simulink model "CM700A_HwTq3Meas"  (R2013b)
settings: Solver=FixedStepDiscrete  SolverMode=SingleTasking  StartTime=0.0  StopTime=1  FixedStep=0.002  RelTol=1e-3
values from neighbouring files (symbols this model uses):
  ELECGLBPRM_HWTQOFFS_HWNWTMTR_F32 = DataDict.Constant    [CM700A_HwTq3Meas_DataDict.m]
  ELECGLBPRM_HWTQSATNLOWRLIM_HWNWTMTR_F32 = DataDict.Constant    [CM700A_HwTq3Meas_DataDict.m]
  ELECGLBPRM_HWTQSATNUPPRLIM_HWNWTMTR_F32 = DataDict.Constant    [CM700A_HwTq3Meas_DataDict.m]
  ELECGLBPRM_HWTQSCA_ULS_F32 = DataDict.Constant    [CM700A_HwTq3Meas_DataDict.m]
  ELECGLBPRM_NOFLT_CNT_U08 = DataDict.Constant    [CM700A_HwTq3Meas_DataDict.m]
  ELECGLBPRM_OFFSTRIMNOTPRFM_CNT_U08 = DataDict.Constant    [CM700A_HwTq3Meas_DataDict.m]
  ELECGLBPRM_PRTCLFLT_CNT_U08 = DataDict.Constant    [CM700A_HwTq3Meas_DataDict.m]
  ELECGLBPRM_SNSRINTFLT_CNT_U08 = DataDict.Constant    [CM700A_HwTq3Meas_DataDict.m]
  GearIdn2 = DataDict.OpSignal    [CM700A_HwTq3Meas_DataDict.m]
  HwTq3MeasHwTq3PrtclFltFailStep = DataDict.Calibration    [CM700A_HwTq3Meas_DataDict.m]
  HwTq3MeasHwTq3PrtclFltPassStep = DataDict.Calibration    [CM700A_HwTq3Meas_DataDict.m]
undefined symbols (not defined in the file or in its folder): NtcNr1, NtcSts1, sigbuilder_block, SigQlfr1
libraries: simulink x22, NxtrNvM x3
(part 1 of 3)
settings Model: RequirementInfo={'doors' '00006115' '1' 'false' 'DOORS Surrogate Item' '' } %GIDa_184d7b6b_0c7e_41d3_b9a0_1a88eb3981d4  reqMgrSettings="100 S'doors','misc'{{S'surrogatepath','savemodel','savesurrogate','updateLinks','doorsLinks2sl','slLinks2Doors','purgeDoors','purgeSimulink','detaillevel','surrogateId','synctime'{{T\"/ESG Group/CM660A_HwTq1Meas\",M[1],M[1],M[0],M[0],M[1],M[0],M[0],M[1],T\"00006115\",T\"\"}},S'mode','pathStorage'{{T\"generic\",T\"modelRelative\"}}}}"  RecordCoverage=on  CovMetricSettings=dcmtrzoiw  CovFilter=CM700A_HwTq3Meas_covfilter  CovHTMLOptions=-sRT=1 -aTS=1 -bRG=1 -bTC=1 -hTR=0 -nFC=0 -scm=1 -bcm=1 -xEv=0  CovModelRefEnable=all  CovExternalEMLEnable=on  Creator=CZ68DS  LastModifiedBy=TZBSJD
settings SolverCC: AutoInsertRateTranBlk=on  InsertRTBMode=Always
settings DataIOCC: LimitDataPoints=off  SaveFormat=Structure  ReturnWorkspaceOutputs=on
settings OptimizationCC: BlockReduction=off  InlineParams=on  ZeroExternalMemoryAtStartup=off  ZeroInternalMemoryAtStartup=off  OptimizeModelRefInitCode=on  LifeSpan=1
settings DebuggingCC: SignalInfNanChecking=error  SignalRangeChecking=warning  UnderspecifiedInitializationDetection=Simplified  SolverPrmCheckMsg=error  InheritedTsInSrcMsg=error  DiscreteInheritContinuousMsg=error  SingleTaskRateTransMsg=error  TasksWithSamePriorityMsg=error  SigSpecEnsureSampleTimeMsg=error  CheckMatrixSingularityMsg=error  ParameterUnderflowMsg=error  ParameterPrecisionLossMsg=error  ParameterTunabilityLossMsg=error  FixptConstUnderflowMsg=warning  FixptConstOverflowMsg=warning  VectorMatrixConversionMsg=error  SignalLabelMismatchMsg=error  UnconnectedInputMsg=error  UnconnectedOutputMsg=error  UnconnectedLineMsg=error  SFcnCompatibilityMsg=error  UniqueDataStoreMsg=warning  BusObjectLabelMismatch=error  RootOutportRequireBusObject=error  AssertControl=DisableAll  ModelReferenceIOMsg=error  ModelReferenceVersionMismatchMessage=warning  ModelReferenceIOMismatchMessage=error  ModelReferenceCSMismatchMessage=warning  ModelReferenceDataLoggingMessage=error  StateNameClashWarn=warning  StrictBusMsg=ErrorOnBusTreatedAsVector  NonBusSignalsTreatedAsBus=error  SFUnexpectedBacktrackingDiag=error  SFInvalidInputDataAccessInChartInitDiag=error  SFNoUnconditionalDefaultTransitionDiag=error  SFTransitionOutsideNaturalParentDiag=error  SFUnconditionalTransitionShadowingDiag=error  SFUndirectedBroadcastEventsDiag=error
settings ModelReferenceCC: ModelReferenceNumInstancesAllowed=Single
settings RTWCC: SystemTargetFile=autosar.tlc  GenCodeOnly=on  TemplateMakefile=ert_default_tmf  Description=AUTOSAR  GenerateReport=on  ProcessScript=autosar_make_rtw_hook  LaunchReport=on
settings CodeAppCC: GenerateComments=off  IgnoreCustomStorageClasses=off  CustomSymbolStrType=$N$R$M  CustomSymbolStrBlkIO=$N$M  SimulinkBlockComments=off
settings STFCustomTargetCC: ParMdlRefBuildCompliant=on  CompOptLevelCompliant=on  IncludeMdlTerminateFcn=off  CombineOutputUpdateFcns=on  SuppressErrorStatus=on  ERTFirstTimeCompliant=on  ERTCustomFileBanners=on  SupportNonFinite=off  SupportComplex=off  SupportContinuousTime=off  SupportNonInlinedSFcns=off  MATLABClassNameForMDSCustomization=Simulink.SoftwareTarget.ERTCustomization  AutosarCompliant=on  GRTInterface=off  SystemTargetFile=autosar.tlc
settings ERTTargetCC: CodeReplacementLibrary=ANSI_C  ConcurrentExecutionCompliant=off  IncludeMdlTerminateFcn=off  SuppressErrorStatus=on  SupportNonFinite=off  SupportComplex=off  ModelStepFunctionPrototypeControlCompliant=off  CPPClassGenCompliant=off  AutosarCompliant=on  InlinedParameterPlacement=NonHierarchical  ERTCustomFileTemplate=example_file_process.tlc  EnableUserReplacementTypes=on

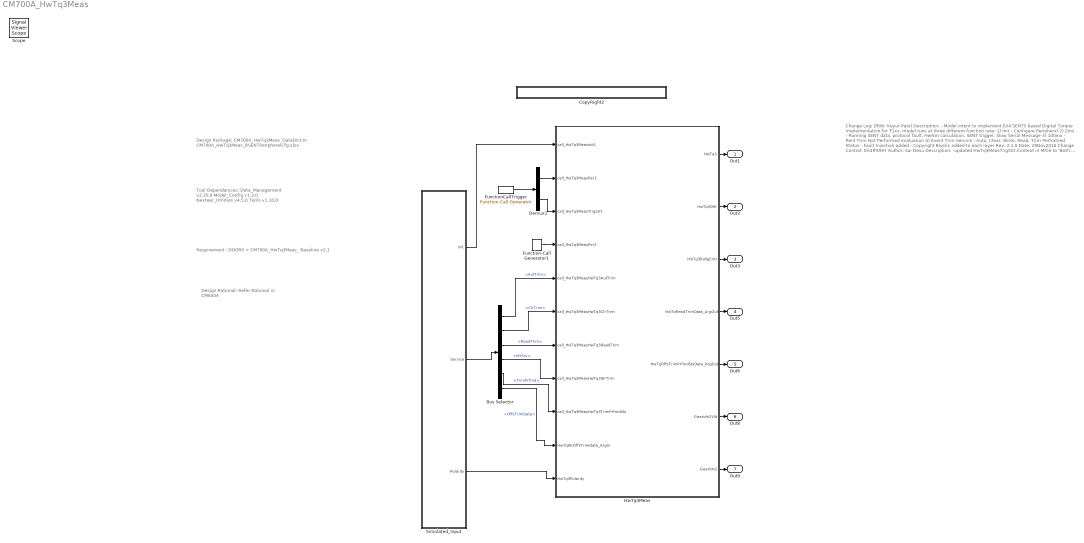
== system CM700A_HwTq3Meas ==
  note: Design Package:
      |
      | CM700A_HwTq3Meas_DataDict.m
      | CM700A_HwTq3Meas_RSENTPeripheralCfg.xlsx
  note: Change Log:
      |
      | DRW: Keyur Patel
      | Description:
      | - Model intent to implement EA4 SENT5 based Digital Torque implementation for T1xx.
      |    model runs at three different function rate:
      |       1) Init - Configure Peripheral
      |       2) 2ms - Running SENT data, protocol fault, HwNm calculation, SENT trigger, Slow Serial Message
      |       3) 100ms - Per3 Trim Not Performed evaluation
      |       4) Event Trim Service - Auto, Clear, Write, Read, Trim Performed Status
      | - Fault Injection added
      | - Copyright Blocks added to each layer
      |
      | Rev: 2.1.0
      | Date: 29Nov2016
      | Change Control: EA4#8597
      | Author: Sai Desu
      | Description:
      | -updated HwTq3MeasTrigStrt.Context in Mfile to 'Both'
      | -Removed Physical Inputs and Outputs from Mfile
      | -Grounded physical inputs and terminated Physical outputs in the model.
      |
      | Rev: 2.0.1
      | Date: 17MAY2016
      | Change Control: EA4#5776
      | Author: K. Patel
      | Description:
      | - GearIdn Uppler Limit and Lower Limit Added
      |
      |
      | Rev: 2.0.0
      | Date: 16MAR2016
      | Change Control: EA4#4736
      | Author: K. Patel
      | Description:
      | - Slow Serial Data Read Added for "C Factor & Bushing" signal read
      | - Timer 2us added before SPCT in NRS check added instead of SYNCM
      | - Refer Red Color High lighted Changes.
      |
      | Rev1.4.0
      | Date: 19JAN2016
      | Change Control #: 3378
      | DRW: K. Patel
      | Description:
      | - Refer Red Color High lighted Changes.
      | - "CM700A_HwTq3Meas_RSENTPeripheralCfg.xlsx" change
      |
      | Rev1.3.0
      | Date: 16DEC2015
      | Change Control #: 3161
      | DRW: K. Patel
      | Description:
      | - Refer Red Color High lighted Changes.
      |
      | Rev: 1.2.0
      | Date: 09OCT2015
      | Change Control #: EA4#1925
      | DRW: K. Patel
      | Description:
      | - Torque Trigger server function, Per3 change to Per2, Missing Message Counter add per1,
      | remove register from "CM700A_HwTq3Meas_RSENTPeripheralCfg.xlsx", change sync time to 16
      |
      | Rev: 1.1.0
      | Date: 31JUL2015
      | Change Control #: WCR-EA4#1232
      | DRW: K. Patel
      | Description:
      | - m file correction, Tick Time change from 1us to 1.2us
      | - Global Constant
      |
      | Rev: 1.0.0
      | Date: 06JUL2015
      | Change Control #: WCR-EA4#1033
      | DRW: K. Patel
      | Description:
      | - Initial Release
      | - Trim Services Added
  note: Tool Dependancies:
      |
      | Data_Management v2.35.0
      | Model_Config v1.3.0
      | Nexteer_Utilities v4.5.0
      | Tools v1.10.0
  note: Requirement :
      |
      | DOORS > CM700A_HwTq3Meas_ Baseline v2.1
  note: Design Rational:
      |
      | Refer Rational in CM650A
  Bus Selector : BusSelector  OutputSignals=AutTrim,ClrTrim,ReadTrim,WrSrv,TrimPrfmd,OffsTrimData
  CopyRight2 : Subsystem  Description=|  mask(Copyright Information){none=on}
      | Copyright info block.                                               
      |                                                                     
      | Place copyright information at the top of every subsystem in design.
      mask prompts: none "No parameters"
      mask help: Place copyright information at the top of every subsystem in design.
      mask Display:
      | NxtrConf = 'Nexteer Confidential';
      | 
      | sys = bdroot; %handle for the current model ("system")
      | first = get_param(sys,'Created');
      | first = first(end-3:end);  %year is last four digits
      | 
      | last = get_param(sys,'LastModifiedDate');
      | if isempty(last)
      |     last = datestr(now,'yyyy');
      | else
      |     last = last(end-3:end);
      | end
      | 
      | if strcmp(first,last)
      |     fprintf('%s -- Copyright %s Nexteer',NxtrConf,first)
      | else
      |     fprintf('%s -- %s%s- %s Nexteer',NxtrConf,char(169),first,last)
      | end
  Demux1 : Demux  Outputs=2
  Function-Call Generator1 : simulink/Ports & Subsystems/Function-Call Generator  sample_time=0.100  numberOfIterations=1
  FunctionCallTrigger : simulink/Ports & Subsystems/Function-Call Generator  RequirementInfo={} %GIDa_461051ca_e299_4da2_91c0_e73e41056377  sample_time=0.002  numberOfIterations=1
  HwTq3Meas : Subsystem  RequirementInfo={} %GIDa_76d712c1_5f1a_450e_83af_7c4f481758f4  Priority=1
      settings: AttributesFormatString=Priority = %<Priority>
  Simulated_Input : Subsystem  Description=Do not Code this block
      settings: AttributesFormatString=%<Description>
  Out1 : Outport
  Out2 : Outport  Port=2
  Out3 : Outport  Port=3
  Out5 : Outport  Port=4
  Out6 : Outport  Port=5
  Out8 : Outport  Port=6
  Out9 : Outport  Port=7
  Scope : SignalViewerScope  IOType=viewer  RefreshTime=0.035000
  wires:
  FunctionCallTrigger/1 -> Demux1/1
  Simulated_Input/3(Polarity) -> HwTq3Meas/11(HwTq3Polarity)
  HwTq3Meas/3(HwTq3RollgCntr) -> Out3/1
  HwTq3Meas/1(HwTq3) -> Out1/1
  HwTq3Meas/2(HwTq3Qlfr) -> Out2/1
  Function-Call Generator1/1 -> HwTq3Meas/4(call_HwTq3MeasPer2)
  Demux1/1 -> HwTq3Meas/2(call_HwTq3MeasPer1)
  Demux1/2 -> HwTq3Meas/3(call_HwTq3MeasTrigStrt)
  Bus Selector/1 -> HwTq3Meas/5(call_HwTq3MeasHwTq3AutTrim)  "<AutTrim>"
  Bus Selector/2 -> HwTq3Meas/6(call_HwTq3MeasHwTq3ClrTrim)  "<ClrTrim>"
  Bus Selector/3 -> HwTq3Meas/7(call_HwTq3MeasHwTq3ReadTrim)  "<ReadTrim>"
  Bus Selector/4 -> HwTq3Meas/8(call_HwTq3MeasHwTq3WrTrim)  "<WrSrv>"
  Bus Selector/5 -> HwTq3Meas/9(call_HwTq3MeasHwTq3TrimPrfmdSts)  "<TrimPrfmd>"
  Bus Selector/6 -> HwTq3Meas/10(HwTqWrOffsTrimData_ArgIn)  "<OffsTrimData>"
  Simulated_Input/1(Init) -> HwTq3Meas/1(call_HwTq3MeasInit1)
  Simulated_Input/2(Service) -> Bus Selector/1
  HwTq3Meas/4(HwTqReadTrimData_ArgOut) -> Out5/1
  HwTq3Meas/5(HwTqOffsTrimPrfmdStsData_ArgOut) -> Out6/1
  HwTq3Meas/6(GearIdn2Vld) -> Out8/1
  HwTq3Meas/7(GearIdn2) -> Out9/1

== system CM700A_HwTq3Meas/CopyRight2 ==

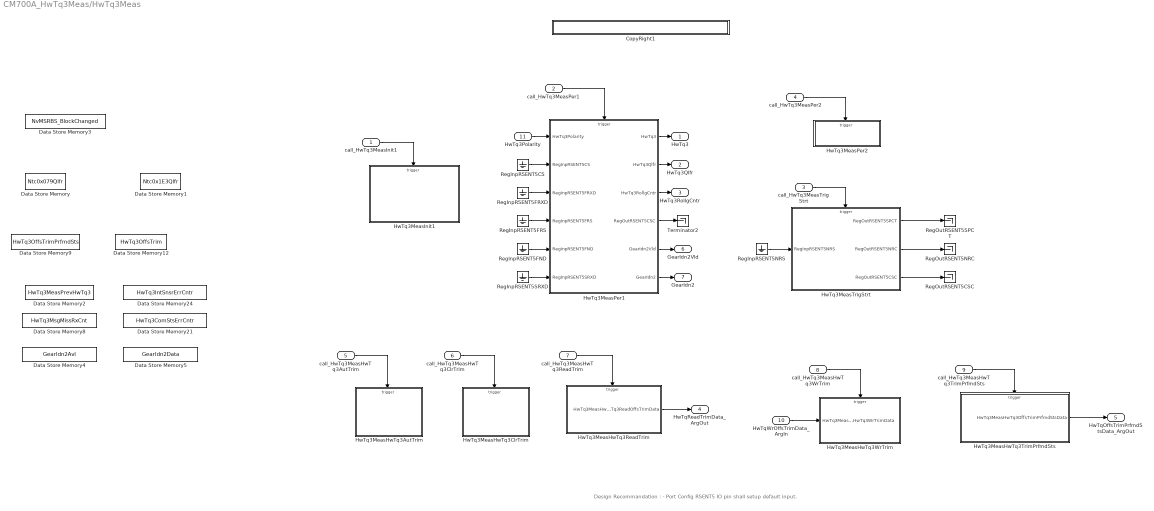
== system CM700A_HwTq3Meas/HwTq3Meas ==
  note: Design Recommandation :
      |
      | - Port Config RSENT5 IO pin shall setup default input.
  call_HwTq3MeasInit1 : Inport
  call_HwTq3MeasPer1 : Inport  Description=2ms  Port=2
      settings: AttributesFormatString=%<Description>
  call_HwTq3MeasTrigStrt : Inport  Description=Event  Port=3
      settings: AttributesFormatString=%<Description>
  call_HwTq3MeasPer2 : Inport  Description=100ms  Port=4
      settings: AttributesFormatString=%<Description>
  call_HwTq3MeasHwTq3AutTrim : Inport  Description=Event  Port=5
      settings: AttributesFormatString=%<Description>
  call_HwTq3MeasHwTq3ClrTrim : Inport  Description=Event  Port=6
      settings: AttributesFormatString=%<Description>
  call_HwTq3MeasHwTq3ReadTrim : Inport  Description=Event  Port=7
      settings: AttributesFormatString=%<Description>
  call_HwTq3MeasHwTq3WrTrim : Inport  Description=Event  Port=8
      settings: AttributesFormatString=%<Description>
  call_HwTq3MeasHwTq3TrimPrfmdSts : Inport  Description=Event  Port=9
      settings: AttributesFormatString=%<Description>
  HwTqWrOffsTrimData_ArgIn : Inport  Port=10
  HwTq3Polarity : Inport  Port=11  OutDataTypeStr=int8
  CopyRight1 : Subsystem  Description=|  mask(Copyright Information){none=on}
      | Copyright info block.                                               
      |                                                                     
      | Place copyright information at the top of every subsystem in design.
      mask prompts: none "No parameters"
      mask help: Place copyright information at the top of every subsystem in design.
      mask Display:
      | NxtrConf = 'Nexteer Confidential';
      | 
      | sys = bdroot; %handle for the current model ("system")
      | first = get_param(sys,'Created');
      | first = first(end-3:end);  %year is last four digits
      | 
      | last = get_param(sys,'LastModifiedDate');
      | if isempty(last)
      |     last = datestr(now,'yyyy');
      | else
      |     last = last(end-3:end);
      | end
      | 
      | if strcmp(first,last)
      |     fprintf('%s -- Copyright %s Nexteer',NxtrConf,first)
      | else
      |     fprintf('%s -- %s%s- %s Nexteer',NxtrConf,char(169),first,last)
      | end
  Data Store Memory12 : DataStoreMemory  DataStoreName=HwTq3OffsTrim  ReadBeforeWriteMsg=warning  WriteAfterWriteMsg=warning  WriteAfterReadMsg=warning
  Data Store Memory2 : DataStoreMemory  DataStoreName=HwTq3MeasPrevHwTq3  ReadBeforeWriteMsg=warning  WriteAfterWriteMsg=warning  WriteAfterReadMsg=warning  StateMustResolveToSignalObject=on
  Data Store Memory21 : DataStoreMemory  DataStoreName=HwTq3ComStsErrCntr  ReadBeforeWriteMsg=warning  WriteAfterWriteMsg=warning  WriteAfterReadMsg=warning  StateMustResolveToSignalObject=on
  Data Store Memory24 : DataStoreMemory  DataStoreName=HwTq3IntSnsrErrCntr  ReadBeforeWriteMsg=warning  WriteAfterWriteMsg=warning  WriteAfterReadMsg=warning  StateMustResolveToSignalObject=on
  Data Store Memory4 : DataStoreMemory  DataStoreName=GearIdn2Avl  ReadBeforeWriteMsg=warning  WriteAfterWriteMsg=warning  WriteAfterReadMsg=warning  StateMustResolveToSignalObject=on
  Data Store Memory5 : DataStoreMemory  DataStoreName=GearIdn2Data  ReadBeforeWriteMsg=warning  WriteAfterWriteMsg=warning  WriteAfterReadMsg=warning  StateMustResolveToSignalObject=on
  Data Store Memory8 : DataStoreMemory  DataStoreName=HwTq3MsgMissRxCnt  ReadBeforeWriteMsg=warning  WriteAfterWriteMsg=warning  WriteAfterReadMsg=warning  StateMustResolveToSignalObject=on
  Data Store Memory9 : DataStoreMemory  DataStoreName=HwTq3OffsTrimPrfmdSts  ReadBeforeWriteMsg=warning  WriteAfterWriteMsg=warning  WriteAfterReadMsg=warning
  Data Store Memory : DataStoreMemory  DataStoreName=Ntc0x079Qlfr  ReadBeforeWriteMsg=warning  WriteAfterWriteMsg=warning  WriteAfterReadMsg=warning  OutDataTypeStr=uint8
      settings: AttributesFormatString=|
      | Simulation Purpose Only.
      | Do Not Code this block
      | Diagnostic Manager Owns this requirement
  Data Store Memory1 : DataStoreMemory  DataStoreName=Ntc0x1E3Qlfr  ReadBeforeWriteMsg=warning  WriteAfterWriteMsg=warning  WriteAfterReadMsg=warning  OutDataTypeStr=uint8
      settings: AttributesFormatString=|
      | Simulation Purpose Only.
      | Do Not Code this block
      | Diagnostic Manager Owns this requirement
  Data Store Memory3 : DataStoreMemory  DataStoreName=NvMSRBS_BlockChanged  ReadBeforeWriteMsg=warning  WriteAfterWriteMsg=warning  WriteAfterReadMsg=warning  OutDataTypeStr=uint8
      settings: AttributesFormatString=|
      | Simulation Purpose Only.
      | Do Not Code this block
      | Diagnostic Manager Owns this requirement
  HwTq3MeasHwTq3AutTrim : Subsystem  RequirementInfo={'linktype_rmi_doors' '0000cf43 (/ESG Group/FDD Module Requirements/EA4 Specific/CM700A_HwTq3Meas)' '#CM700A_56' 'true' 'REQ: CM700A_56' '' } %GIDa_78a0150d_b2b2_4893_8cf0_7a267cd87682  Priority=10  TreatAsAtomicUnit=on
      settings: AttributesFormatString=Priority=%<Priority>
  HwTq3MeasHwTq3ClrTrim : Subsystem  RequirementInfo={'linktype_rmi_doors' '0000cf43 (/ESG Group/FDD Module Requirements/EA4 Specific/CM700A_HwTq3Meas)' '#CM700A_54' 'true' 'REQ: CM700A_54' '' } %GIDa_9d8bf3ad_e540_4a5e_ad4c_eb940ac157ad  Priority=10  TreatAsAtomicUnit=on
      settings: AttributesFormatString=Priority=%<Priority>
  HwTq3MeasHwTq3ReadTrim : Subsystem  RequirementInfo={'linktype_rmi_doors' '0000cf43 (/ESG Group/FDD Module Requirements/EA4 Specific/CM700A_HwTq3Meas)' '#CM700A_52' 'true' 'REQ: CM700A_52' '' } %GIDa_4c78535b_9e38_436f_a670_46438fd62cfe  Priority=10  TreatAsAtomicUnit=on
      settings: AttributesFormatString=Priority=%<Priority>
  HwTq3MeasHwTq3TrimPrfmdSts : Subsystem  RequirementInfo={'linktype_rmi_doors' '0000cf43 (/ESG Group/FDD Module Requirements/EA4 Specific/CM700A_HwTq3Meas)' '#CM700A_53' 'true' 'REQ: CM700A_53' '' } %GIDa_05e70ef2_f8d5_471c_a4a3_b95d94c92180  Priority=10  TreatAsAtomicUnit=on
      settings: AttributesFormatString=Priority=%<Priority>
  HwTq3MeasHwTq3WrTrim : Subsystem  RequirementInfo={'linktype_rmi_doors' '0000cf43 (/ESG Group/FDD Module Requirements/EA4 Specific/CM700A_HwTq3Meas)' '#CM700A_55' 'true' 'REQ: CM700A_55' '' } %GIDa_58f23a20_9e17_4252_b727_77362ca5c7be  Priority=10  TreatAsAtomicUnit=on
      settings: AttributesFormatString=Priority=%<Priority>
  HwTq3MeasInit1 : Subsystem  TreatAsAtomicUnit=on
  HwTq3MeasPer1 : Subsystem  RequirementInfo={'linktype_rmi_doors' '0000cf43 (/ESG Group/FDD Module Requirements/EA4 Specific/CM700A_HwTq3Meas)' '#CM700A_39' 'true' 'REQ: CM700A_39' '' } %GIDa_31b3da74_5937_4fb2_b915_5c5c5e5711e7  TreatAsAtomicUnit=on
  HwTq3MeasPer2 : Subsystem  RequirementInfo={'linktype_rmi_doors' '0000cf43 (/ESG Group/FDD Module Requirements/EA4 Specific/CM700A_HwTq3Meas)' '#CM700A_61' 'true' 'REQ: CM700A_61' '' } %GIDa_c89b04b6_b4c1_41bf_b3f8_efad30b9fb82  Priority=8  TreatAsAtomicUnit=on
      settings: AttributesFormatString=Priority=%<Priority>
  HwTq3MeasTrigStrt : Subsystem  RequirementInfo={'linktype_rmi_doors' '0000cf43 (/ESG Group/FDD Module Requirements/EA4 Specific/CM700A_HwTq3Meas)' '#CM700A_33' 'true' 'REQ: CM700A_33' '' } %GIDa_ac2e4248_233e_47e7_8dc6_e55969fb5c4e  TreatAsAtomicUnit=on
  RegInpRSENT5CS : Ground
  RegInpRSENT5FND : Ground
  RegInpRSENT5FRS : Ground
  RegInpRSENT5FRXD : Ground
  RegInpRSENT5NRS : Ground
  RegInpRSENT5SRXD : Ground
  RegOutRSENT5CSC : Terminator
  RegOutRSENT5NRC : Terminator
  RegOutRSENT5SPCT : Terminator
  Terminator2 : Terminator
  HwTq3 : Outport
  HwTq3Qlfr : Outport  Port=2
  HwTq3RollgCntr : Outport  Port=3
  HwTqReadTrimData_ArgOut : Outport  Port=4
  HwTqOffsTrimPrfmdStsData_ArgOut : Outport  Port=5
  GearIdn2Vld : Outport  Port=6
  GearIdn2 : Outport  Port=7
  wires:
  call_HwTq3MeasPer1/1 -> HwTq3MeasPer1/Trigger
  call_HwTq3MeasInit1/1 -> HwTq3MeasInit1/Trigger
  HwTq3MeasPer1/1(HwTq3) -> HwTq3/1
  HwTq3MeasPer1/2(HwTq3Qlfr) -> HwTq3Qlfr/1
  HwTq3MeasPer1/3(HwTq3RollgCntr) -> HwTq3RollgCntr/1
  call_HwTq3MeasTrigStrt/1 -> HwTq3MeasTrigStrt/Trigger
  HwTq3Polarity/1 -> HwTq3MeasPer1/1(HwTq3Polarity)
  HwTq3MeasTrigStrt/1(RegOutRSENT5SPCT) -> RegOutRSENT5SPCT/1
  call_HwTq3MeasHwTq3AutTrim/1 -> HwTq3MeasHwTq3AutTrim/Trigger
  call_HwTq3MeasHwTq3ClrTrim/1 -> HwTq3MeasHwTq3ClrTrim/Trigger
  call_HwTq3MeasHwTq3ReadTrim/1 -> HwTq3MeasHwTq3ReadTrim/Trigger
  call_HwTq3MeasHwTq3WrTrim/1 -> HwTq3MeasHwTq3WrTrim/Trigger
  call_HwTq3MeasHwTq3TrimPrfmdSts/1 -> HwTq3MeasHwTq3TrimPrfmdSts/Trigger
  HwTqWrOffsTrimData_ArgIn/1 -> HwTq3MeasHwTq3WrTrim/1(HwTq3MeasHwTq3WrTrimData)
  HwTq3MeasHwTq3ReadTrim/1(HwTq3MeasHwTq3ReadOffsTrimData) -> HwTqReadTrimData_ArgOut/1
  HwTq3MeasHwTq3TrimPrfmdSts/1(HwTq3MeasHwTq3OffsTrimPrfmdStsData) -> HwTqOffsTrimPrfmdStsData_ArgOut/1
  call_HwTq3MeasPer2/1 -> HwTq3MeasPer2/Trigger
  RegInpRSENT5CS/1 -> HwTq3MeasPer1/2(RegInpRSENT5CS)
  RegInpRSENT5FRXD/1 -> HwTq3MeasPer1/3(RegInpRSENT5FRXD)
  RegInpRSENT5FRS/1 -> HwTq3MeasPer1/4(RegInpRSENT5FRS)
  RegInpRSENT5FND/1 -> HwTq3MeasPer1/5(RegInpRSENT5FND)
  HwTq3MeasTrigStrt/2(RegOutRSENT5NRC) -> RegOutRSENT5NRC/1
  HwTq3MeasTrigStrt/3(RegOutRSENT5CSC) -> RegOutRSENT5CSC/1
  RegInpRSENT5NRS/1 -> HwTq3MeasTrigStrt/1(RegInpRSENT5NRS)
  HwTq3MeasPer1/4(RegOutRSENT5CSC) -> Terminator2/1
  RegInpRSENT5SRXD/1 -> HwTq3MeasPer1/6(RegInpRSENT5SRXD)
  HwTq3MeasPer1/5(GearIdn2Vld) -> GearIdn2Vld/1
  HwTq3MeasPer1/6(GearIdn2) -> GearIdn2/1

== system CM700A_HwTq3Meas/Simulated_Input ==
  Bus Creator : BusCreator  Inputs=6
  CopyRight2 : Subsystem  Description=|  mask(Copyright Information){none=on}
      | Copyright info block.                                               
      |                                                                     
      | Place copyright information at the top of every subsystem in design.
      mask prompts: none "No parameters"
      mask help: Place copyright information at the top of every subsystem in design.
      mask Display:
      | NxtrConf = 'Nexteer Confidential';
      | 
      | sys = bdroot; %handle for the current model ("system")
      | first = get_param(sys,'Created');
      | first = first(end-3:end);  %year is last four digits
      | 
      | last = get_param(sys,'LastModifiedDate');
      | if isempty(last)
      |     last = datestr(now,'yyyy');
      | else
      |     last = last(end-3:end);
      | end
      | 
      | if strcmp(first,last)
      |     fprintf('%s -- Copyright %s Nexteer',NxtrConf,first)
      | else
      |     fprintf('%s -- %s%s- %s Nexteer',NxtrConf,char(169),first,last)
      | end
  Data Type Conversion1 : DataTypeConversion  OutDataTypeStr=int8
  Data Type Conversion6 : DataTypeConversion  OutDataTypeStr=single
  Rate Transition : RateTransition
  Signal Builder : Subsystem  Tag=STV Subsys  LoadFcn=sigbuilder_block('load');  StartFcn=sigbuilder_block('start');  StopFcn=sigbuilder_block('stop');  ClipboardFcn=sigbuilder_block('clipboard');  mask(Sigbuilder block){}
      mask help: Simulink:masks:SigbuilderBlock_MD
      mask init:
      | if ~strcmp(get_param(bdroot(gcbh),'SimulationStatus'),'stopped') tuvar = sigbuilder_block('maskInit'); end
      settings: CopyFcn=sigbuilder_block('copy');  DeleteFcn=sigbuilder_block('delete');  ModelCloseFcn=sigbuilder_block('modelClose');  PreSaveFcn=sigbuilder_block('preSave');  PauseFcn=sigbuilder_block('pause');  ContinueFcn=sigbuilder_block('continue');  NameChangeFcn=sigbuilder_block('namechange');  OpenFcn=sigbuilder_block('open',[56.4828 0 967.655 519.517 ]);  CloseFcn=sigbuilder_block('close');
      mask Display: plot(0, 0, 100, 100,[2, 2, 32, 32, 2], [68, 8, 8, 68, 68],[32, 2], [38, 38], [32, 19, 2],[53, 60, 44], [32, 17, 17, 2],[16, 16, 31, 31]);txt = getActiveGroup(gcbh);text(2, 100, txt,'verticalAlignment', 'top');
  Init : Outport
  Service : Outport  Port=2
  Polarity : Outport  Port=3
  wires:
  Signal Builder/8(Polarity) -> Data Type Conversion1/1  "Polarity"
  Signal Builder/1(InitTrg) -> Init/1
  Signal Builder/7(HwTqOffsTrimData) -> Data Type Conversion6/1
  Signal Builder/6(TrimPrfmdStsSrv) -> Bus Creator/5  "TrimPrfmd"
  Signal Builder/5(WrSrv) -> Bus Creator/4  "WrSrv"
  Signal Builder/4(ReadTrimSrv) -> Bus Creator/3  "ReadTrim"
  Signal Builder/3(ClearTrimSrv) -> Bus Creator/2  "ClrTrim"
  Signal Builder/2(AutTrimSrv) -> Bus Creator/1  "AutTrim"
  Bus Creator/1 -> Service/1
  Data Type Conversion1/1 -> Rate Transition/1
  Rate Transition/1 -> Polarity/1
  Data Type Conversion6/1 -> Bus Creator/6  "OffsTrimData"

== system CM700A_HwTq3Meas/HwTq3Meas/CopyRight1 ==

== system CM700A_HwTq3Meas/HwTq3Meas/HwTq3MeasHwTq3AutTrim ==
  function : TriggerPort
  CopyRight2 : Subsystem  Description=|  mask(Copyright Information){none=on}
      | Copyright info block.                                               
      |                                                                     
      | Place copyright information at the top of every subsystem in design.
      mask prompts: none "No parameters"
      mask help: Place copyright information at the top of every subsystem in design.
      mask Display:
      | NxtrConf = 'Nexteer Confidential';
      | 
      | sys = bdroot; %handle for the current model ("system")
      | first = get_param(sys,'Created');
      | first = first(end-3:end);  %year is last four digits
      | 
      | last = get_param(sys,'LastModifiedDate');
      | if isempty(last)
      |     last = datestr(now,'yyyy');
      | else
      |     last = last(end-3:end);
      | end
      | 
      | if strcmp(first,last)
      |     fprintf('%s -- Copyright %s Nexteer',NxtrConf,first)
      | else
      |     fprintf('%s -- %s%s- %s Nexteer',NxtrConf,char(169),first,last)
      | end
  NVM Shadow RAM : DataStoreWrite  RequirementInfo={} %GIDa_691c2588_2b45_48b9_9733_fd18f25444bb  DataStoreName=HwTq3OffsTrim
  NVM1 Shadow RAM : DataStoreWrite  RequirementInfo={'linktype_rmi_doors' '0000cf43 (/ESG Group/FDD Module Requirements/EA4 Specific/CM700A_HwTq3Meas)' '#CM700A_50' 'true' 'REQ: CM700A_50' '' } %GIDa_8dfe2b68_c9bd_4b5f_9a85_4945a725dea6  DataStoreName=HwTq3OffsTrimPrfmdSts
  PIM : DataStoreRead  RequirementInfo={} %GIDa_7720d852_cab6_4ee8_822b_ee5ddb596286  Priority=10  DataStoreName=HwTq3MeasPrevHwTq3
      settings: AttributesFormatString=Priority=%<Priority>
  Set : Constant
  Set Ram Block Status : NxtrNvM/Set Ram Block Status  FuncName=Set Ram Block Status  NvMBlockName=HwTq3Offs  VoidFuncRtn=on  BlockChanged_DSN=NvMSRBS_BlockChanged  Return_DSN=NvMSRBS_Return
      settings: AttributesFormatString=%<FuncName>
  Set3 : Constant  OutDataTypeStr=uint8
  wires:
  PIM/1 -> NVM Shadow RAM/1
  Set/1 -> NVM1 Shadow RAM/1
  Set3/1 -> Set Ram Block Status/1

== system CM700A_HwTq3Meas/HwTq3Meas/HwTq3MeasHwTq3ClrTrim ==
  function : TriggerPort
  Clear1 : Constant  Value=0  OutDataTypeStr=single
  Clear2 : Constant  Value=0
  CopyRight2 : Subsystem  Description=|  mask(Copyright Information){none=on}
      | Copyright info block.                                               
      |                                                                     
      | Place copyright information at the top of every subsystem in design.
      mask prompts: none "No parameters"
      mask help: Place copyright information at the top of every subsystem in design.
      mask Display:
      | NxtrConf = 'Nexteer Confidential';
      | 
      | sys = bdroot; %handle for the current model ("system")
      | first = get_param(sys,'Created');
      | first = first(end-3:end);  %year is last four digits
      | 
      | last = get_param(sys,'LastModifiedDate');
      | if isempty(last)
      |     last = datestr(now,'yyyy');
      | else
      |     last = last(end-3:end);
      | end
      | 
      | if strcmp(first,last)
      |     fprintf('%s -- Copyright %s Nexteer',NxtrConf,first)
      | else
      |     fprintf('%s -- %s%s- %s Nexteer',NxtrConf,char(169),first,last)
      | end
  NVM Shadow RAM : DataStoreWrite  RequirementInfo={} %GIDa_c01938bd_873a_4f20_8aad_b7368db2e426  DataStoreName=HwTq3OffsTrim
  NVM1 Shadow RAM : DataStoreWrite  RequirementInfo={'linktype_rmi_doors' '0000cf43 (/ESG Group/FDD Module Requirements/EA4 Specific/CM700A_HwTq3Meas)' '#CM700A_50' 'true' 'REQ: CM700A_50' '' } %GIDa_7e661117_be14_43c5_b4c7_51bd14c3b186  DataStoreName=HwTq3OffsTrimPrfmdSts
  Set Ram Block Status : NxtrNvM/Set Ram Block Status  FuncName=Set Ram Block Status  NvMBlockName=HwTq3Offs  VoidFuncRtn=on  BlockChanged_DSN=NvMSRBS_BlockChanged  Return_DSN=NvMSRBS_Return
      settings: AttributesFormatString=%<FuncName>
  Set3 : Constant  OutDataTypeStr=uint8
  wires:
  Clear1/1 -> NVM Shadow RAM/1
  Clear2/1 -> NVM1 Shadow RAM/1
  Set3/1 -> Set Ram Block Status/1

== system CM700A_HwTq3Meas/HwTq3Meas/HwTq3MeasHwTq3ReadTrim ==
  function : TriggerPort
  CopyRight2 : Subsystem  Description=|  mask(Copyright Information){none=on}
      | Copyright info block.                                               
      |                                                                     
      | Place copyright information at the top of every subsystem in design.
      mask prompts: none "No parameters"
      mask help: Place copyright information at the top of every subsystem in design.
      mask Display:
      | NxtrConf = 'Nexteer Confidential';
      | 
      | sys = bdroot; %handle for the current model ("system")
      | first = get_param(sys,'Created');
      | first = first(end-3:end);  %year is last four digits
      | 
      | last = get_param(sys,'LastModifiedDate');
      | if isempty(last)
      |     last = datestr(now,'yyyy');
      | else
      |     last = last(end-3:end);
      | end
      | 
      | if strcmp(first,last)
      |     fprintf('%s -- Copyright %s Nexteer',NxtrConf,first)
      | else
      |     fprintf('%s -- %s%s- %s Nexteer',NxtrConf,char(169),first,last)
      | end
  NVM Shadow RAM : DataStoreRead  DataStoreName=HwTq3OffsTrim
  HwTq3MeasHwTq3ReadOffsTrimData : Outport
  wires:
  NVM Shadow RAM/1 -> HwTq3MeasHwTq3ReadOffsTrimData/1

== system CM700A_HwTq3Meas/HwTq3Meas/HwTq3MeasHwTq3TrimPrfmdSts ==
  function : TriggerPort
  CopyRight2 : Subsystem  Description=|  mask(Copyright Information){none=on}
      | Copyright info block.                                               
      |                                                                     
      | Place copyright information at the top of every subsystem in design.
      mask prompts: none "No parameters"
      mask help: Place copyright information at the top of every subsystem in design.
      mask Display:
      | NxtrConf = 'Nexteer Confidential';
      | 
      | sys = bdroot; %handle for the current model ("system")
      | first = get_param(sys,'Created');
      | first = first(end-3:end);  %year is last four digits
      | 
      | last = get_param(sys,'LastModifiedDate');
      | if isempty(last)
      |     last = datestr(now,'yyyy');
      | else
      |     last = last(end-3:end);
      | end
      | 
      | if strcmp(first,last)
      |     fprintf('%s -- Copyright %s Nexteer',NxtrConf,first)
      | else
      |     fprintf('%s -- %s%s- %s Nexteer',NxtrConf,char(169),first,last)
      | end
  Data Store Read1 : DataStoreRead  DataStoreName=HwTq3OffsTrimPrfmdSts
  HwTq3MeasHwTq3OffsTrimPrfmdStsData : Outport
  wires:
  Data Store Read1/1 -> HwTq3MeasHwTq3OffsTrimPrfmdStsData/1

== system CM700A_HwTq3Meas/HwTq3Meas/HwTq3MeasHwTq3WrTrim ==
  HwTq3MeasHwTq3WrTrimData : Inport
  function : TriggerPort
  CopyRight2 : Subsystem  Description=|  mask(Copyright Information){none=on}
      | Copyright info block.                                               
      |                                                                     
      | Place copyright information at the top of every subsystem in design.
      mask prompts: none "No parameters"
      mask help: Place copyright information at the top of every subsystem in design.
      mask Display:
      | NxtrConf = 'Nexteer Confidential';
      | 
      | sys = bdroot; %handle for the current model ("system")
      | first = get_param(sys,'Created');
      | first = first(end-3:end);  %year is last four digits
      | 
      | last = get_param(sys,'LastModifiedDate');
      | if isempty(last)
      |     last = datestr(now,'yyyy');
      | else
      |     last = last(end-3:end);
      | end
      | 
      | if strcmp(first,last)
      |     fprintf('%s -- Copyright %s Nexteer',NxtrConf,first)
      | else
      |     fprintf('%s -- %s%s- %s Nexteer',NxtrConf,char(169),first,last)
      | end
  NVM Shadow RAM : DataStoreWrite  RequirementInfo={} %GIDa_1659f01a_6b97_4ff1_afb0_e4ba99927e44  DataStoreName=HwTq3OffsTrim
  NVM1 Shadow RAM : DataStoreWrite  RequirementInfo={'linktype_rmi_doors' '0000cf43 (/ESG Group/FDD Module Requirements/EA4 Specific/CM700A_HwTq3Meas)' '#CM700A_50' 'true' 'REQ: CM700A_50' '' } %GIDa_340e34c7_c59a_43cb_a8d9_5aafb58ec96b  DataStoreName=HwTq3OffsTrimPrfmdSts
  Set : Constant
  Set Ram Block Status : NxtrNvM/Set Ram Block Status  FuncName=Set Ram Block Status  NvMBlockName=HwTq3Offs  VoidFuncRtn=on  BlockChanged_DSN=NvMSRBS_BlockChanged  Return_DSN=NvMSRBS_Return
      settings: AttributesFormatString=%<FuncName>
  Set3 : Constant  OutDataTypeStr=uint8
  wires:
  Set/1 -> NVM1 Shadow RAM/1
  HwTq3MeasHwTq3WrTrimData/1 -> NVM Shadow RAM/1
  Set3/1 -> Set Ram Block Status/1

== system CM700A_HwTq3Meas/HwTq3Meas/HwTq3MeasInit1 ==
  note: Follow below steps in same order:
      |
      | 1. Enable Configuration mode, RSENT5MDC.OMC = 1U
      | 2. Verify whether peripheral is in Configuration mode RSENT5MST.OMS ==1U and wait till 2us* ,it is in configuration mode
      | 3. Configure the SENT Register as per  "CM700A_HwTq3Meas_RSENTPeripheralCfg.xlsx"
      | 4. Enable Operation active mode, RSENT5MDC.OMC = 5U
      | 5. Verify whether peripheral is in Opertation active mode RSENT5MST.OMS ==5U and wait till 2us* ,it is in Opertation active mode
      | 6. Client Call "IoHwAb_SetFctPrphlHwTq3"- Port Configuration shall change to output in alternate mode from default input for RSENT5 SPCO IO pin.
      |
      | Note: * - actual minimum is 150ns as per Scott Winder email from Renesas
  function : TriggerPort  TriggerType=falling
  CopyRight2 : Subsystem  Description=|  mask(Copyright Information){none=on}
      | Copyright info block.                                               
      |                                                                     
      | Place copyright information at the top of every subsystem in design.
      mask prompts: none "No parameters"
      mask help: Place copyright information at the top of every subsystem in design.
      mask Display:
      | NxtrConf = 'Nexteer Confidential';
      | 
      | sys = bdroot; %handle for the current model ("system")
      | first = get_param(sys,'Created');
      | first = first(end-3:end);  %year is last four digits
      | 
      | last = get_param(sys,'LastModifiedDate');
      | if isempty(last)
      |     last = datestr(now,'yyyy');
      | else
      |     last = last(end-3:end);
      | end
      | 
      | if strcmp(first,last)
      |     fprintf('%s -- Copyright %s Nexteer',NxtrConf,first)
      | else
      |     fprintf('%s -- %s%s- %s Nexteer',NxtrConf,char(169),first,last)
      | end
  GetRefTmr1MicroSec32bit : Subsystem
      settings: AttributesFormatString=Client Call : Start Time
  GetTiSpan1MicroSec32bit : Subsystem
  IoHwAb_SetFctPrphlHwTq3 : Subsystem
  Terminator1 : Terminator
  wires:
  GetRefTmr1MicroSec32bit/1(RefTmr) -> GetTiSpan1MicroSec32bit/1(RefTmr)
  GetTiSpan1MicroSec32bit/1(TiSpan) -> Terminator1/1

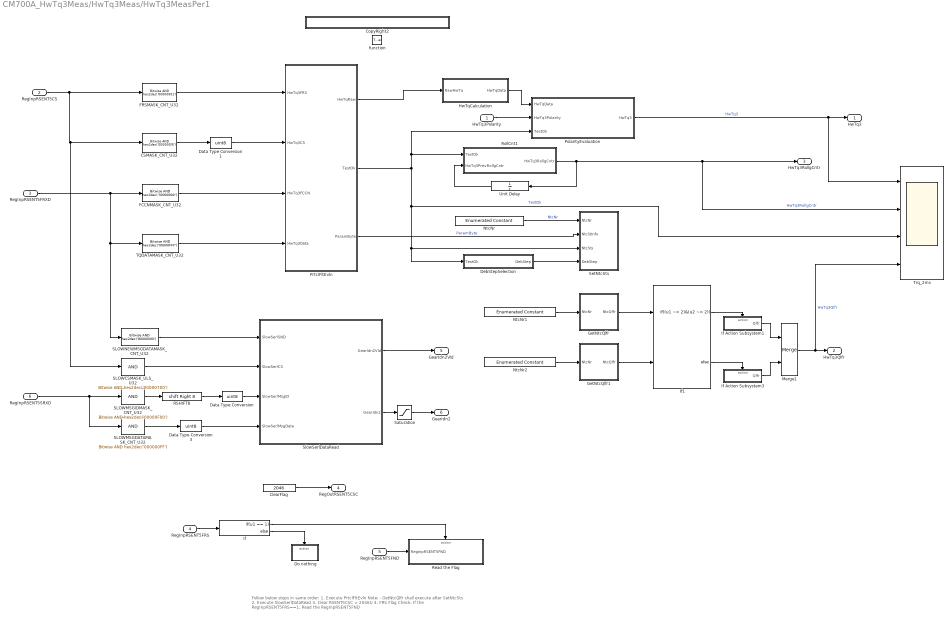
== system CM700A_HwTq3Meas/HwTq3Meas/HwTq3MeasPer1 ==
  note: Follow below steps in same order:
      |
      | 1. Execute PrtclFltEvln
      | Note: - GetNtcQlfr shall execute after SetNtcSts
      | 2. Execute SlowSerlDataRead
      | 3. Clear RSENT5CSC = 2046U
      | 4. FRS Flag Check: If the RegInpRSENT5FRS==1,  Read the RegInpRSENT5FND
  HwTq3Polarity : Inport
  RegInpRSENT5CS : Inport  Port=2
  RegInpRSENT5FRXD : Inport  Port=3
  RegInpRSENT5FRS : Inport  Port=4
  RegInpRSENT5FND : Inport  Port=5
  RegInpRSENT5SRXD : Inport  Port=6
  function : TriggerPort  TriggerType=function-call
  CSMASK_CNT_U32 : simulink/Logic and Bit Operations/Bitwise Operator  logicop=AND  UseBitMask=on  BitMask=hex2dec('000000FE')  BitMaskRealWorld=Stored Integer
  ClearFlag : Constant  RequirementInfo={} %GIDa_f85a4098_a822_4f75_a0b4_b2fef5bc9e6f  Value=2046  OutDataTypeStr=uint16
  CopyRight2 : Subsystem  Description=|  mask(Copyright Information){none=on}
      | Copyright info block.                                               
      |                                                                     
      | Place copyright information at the top of every subsystem in design.
      mask prompts: none "No parameters"
      mask help: Place copyright information at the top of every subsystem in design.
      mask Display:
      | NxtrConf = 'Nexteer Confidential';
      | 
      | sys = bdroot; %handle for the current model ("system")
      | first = get_param(sys,'Created');
      | first = first(end-3:end);  %year is last four digits
      | 
      | last = get_param(sys,'LastModifiedDate');
      | if isempty(last)
      |     last = datestr(now,'yyyy');
      | else
      |     last = last(end-3:end);
      | end
      | 
      | if strcmp(first,last)
      |     fprintf('%s -- Copyright %s Nexteer',NxtrConf,first)
      | else
      |     fprintf('%s -- %s%s- %s Nexteer',NxtrConf,char(169),first,last)
      | end
  Data Type Conversion : DataTypeConversion  OutDataTypeStr=uint8
  Data Type Conversion1 : DataTypeConversion  OutDataTypeStr=uint8
  Data Type Conversion3 : DataTypeConversion  OutDataTypeStr=uint8
  DebStepSelection : Subsystem
  Do nothing : Subsystem  RequirementInfo={} %GIDa_36aa72da_c0b3_4756_827c_f0dd9940ca90  TreatAsAtomicUnit=on
  FCCNMASK_CNT_U32 : simulink/Logic and Bit Operations/Bitwise Operator  logicop=AND  UseBitMask=on  BitMask=hex2dec('30000000')  BitMaskRealWorld=Stored Integer
  FRSMASK_CNT_U32 : simulink/Logic and Bit Operations/Bitwise Operator  logicop=AND  UseBitMask=on  BitMask=hex2dec('00000001')  BitMaskRealWorld=Stored Integer
  GetNtcQlfr : Subsystem
  GetNtcQlfr1 : Subsystem
  HwTqCalculation : Subsystem
  If : If  RequirementInfo={} %GIDa_9a3999db_ec42_4cbc_a179_526d044a0c5a  IfExpression=u1 == 1
  If Action Subsystem1 : Subsystem  TreatAsAtomicUnit=on
  If Action Subsystem3 : Subsystem  TreatAsAtomicUnit=on
  If1 : If  NumInputs=2  IfExpression=(u1 ~= 2)&(u2 ~= 2)
  Merge1 : Merge
  NtcNr : simulink/Sources/Enumerated Constant  OutDataTypeStr=Enum: NtcNr1  Value=NtcNr1.NTCNR_0X079  SampleTime=inf
  NtcNr1 : simulink/Sources/Enumerated Constant  OutDataTypeStr=Enum: NtcNr1  Value=NtcNr1.NTCNR_0X079  SampleTime=inf
  NtcNr2 : simulink/Sources/Enumerated Constant  OutDataTypeStr=Enum: NtcNr1  Value=NtcNr1.NTCNR_0X1E3  SampleTime=inf
  PolarityEvaluation : Subsystem  RequirementInfo={'linktype_rmi_doors' '0000cf43 (/ESG Group/FDD Module Requirements/EA4 Specific/CM700A_HwTq3Meas)' '#CM700A_29' 'true' 'REQ: CM700A_29' '' ; 'linktype_rmi_doors' '0000cf43 (/ESG Group/FDD Module Requirements/EA4 Specific/CM700A_HwTq3Meas)' '#CM700A_32' 'true' 'REQ: CM700A_32' '' } %GIDa_7dd0f124_da9d_41af_bfd5_c8f0b8205e28
  PrtclFltEvln : Subsystem  RequirementInfo={'doors' '00006115' '16' 'false' 'DOORS Surrogate Item' '' ; 'linktype_rmi_doors' '0000cf43 (/ESG Group/FDD Module Requirements/EA4 Specific/CM700A_HwTq3Meas)' '#CM700A_27' 'true' 'REQ: CM700A_27' '' } %GIDa_9ddede9b_2ee1_447b_ab8b_835557d5d4fb
  RSHIFT8 : ArithShift  BitShiftNumber=8  BitShiftDirection=Right
  Read the Flag : Subsystem  RequirementInfo={} %GIDa_8292da39_c813_49b3_bba8_7ea1e085c113  TreatAsAtomicUnit=on
  RollCnt1 : Stateflow chart  RequirementInfo={} %GIDa_be1c412e_1791_4e7e_9b3e_cc09ba9a6629  TreatAsAtomicUnit=on
  SLOWCSMASK_ULS_U32 : simulink/Logic and Bit Operations/Bitwise Operator  logicop=AND  UseBitMask=on  BitMask=hex2dec('00000700')  BitMaskRealWorld=Stored Integer
  SLOWMSGDATAMASK_CNT_U32 : simulink/Logic and Bit Operations/Bitwise Operator  logicop=AND  UseBitMask=on  BitMask=hex2dec('000000FF')  BitMaskRealWorld=Stored Integer
  SLOWMSGIDMASK_CNT_U32 : simulink/Logic and Bit Operations/Bitwise Operator  logicop=AND  UseBitMask=on  BitMask=hex2dec('00000F00')  BitMaskRealWorld=Stored Integer
  SLOWNEWMSGDATAMASK_CNT_U32 : simulink/Logic and Bit Operations/Bitwise Operator  logicop=AND  UseBitMask=on  BitMask=hex2dec('80000000')  BitMaskRealWorld=Stored Integer
  Saturation : Saturate  UpperLimit=GearIdn2.EngMax  LowerLimit=GearIdn2.EngMin
      settings: AttributesFormatString=|
      | %<LowerLimit>
      | %<UpperLimit>
  SetNtcSts : Subsystem  RequirementInfo={'linktype_rmi_doors' '0000cf43 (/ESG Group/FDD Module Requirements/EA4 Specific/CM700A_HwTq3Meas)' '#CM700A_38' 'true' 'REQ: CM700A_38' '' } %GIDa_7c28da3a_b49c_4a2c_9776_430afb4b2413
  SlowSerlDataRead : Subsystem  RequirementInfo={'linktype_rmi_doors' '0000cf43 (/ESG Group/FDD Module Requirements/EA4 Specific/CM700A_HwTq3Meas)' '#CM700A_66' 'true' 'REQ: CM700A_66' '' } %GIDa_a534ff24_7731_4575_902d_df9a309aff98
  TQDATAMASK_CNT_U32 : simulink/Logic and Bit Operations/Bitwise Operator  logicop=AND  UseBitMask=on  BitMask=hex2dec('00000FFF')  BitMaskRealWorld=Stored Integer
  Trq_2ms : Scope  NumInputPorts=4
      settings: TimeRange=20  YMin=-10~0~1.9~0.95  YMax=10~275~2.1~1.05  SaveName=ScopeData3
  Unit Delay : UnitDelay  SampleTime=-1  StateName=HwTq3MeasPrevRollgCntr  StateMustResolveToSignalObject=on
      settings: AttributesFormatString=%<StateName>
  HwTq3 : Outport  RequirementInfo={} %GIDa_3b2abd0f_dff5_44f3_b788_adb2172836f5
  HwTq3Qlfr : Outport  RequirementInfo={'linktype_rmi_doors' '0000cf43 (/ESG Group/FDD Module Requirements/EA4 Specific/CM700A_HwTq3Meas)' '#CM700A_30' 'true' 'REQ: CM700A_30' '' } %GIDa_5eff5979_1038_44df_a727_ac7fcfb158b0  Port=2
  HwTq3RollgCntr : Outport  RequirementInfo={'linktype_rmi_doors' '0000cf43 (/ESG Group/FDD Module Requirements/EA4 Specific/CM700A_HwTq3Meas)' '#CM700A_31' 'true' 'REQ: CM700A_31' '' } %GIDa_de83414f_64c7_40b0_8047_6b8baba686d2  Port=3
  RegOutRSENT5CSC : Outport  Port=4
  GearIdn2Vld : Outport  RequirementInfo={} %GIDa_d279c553_77c2_4307_9c21_10957e80324d  Port=5
  GearIdn2 : Outport  RequirementInfo={} %GIDa_0355680d_a243_40f6_8530_f1f9bdf0d0ac  Port=6
  wires:
  PrtclFltEvln/1(HwTqRaw) -> HwTqCalculation/1(RawHwTq)
  HwTqCalculation/1(HwTqData) -> PolarityEvaluation/1(HwTqData)
  PrtclFltEvln/2(TestOk) -> PolarityEvaluation/3(TestOk), RollCnt1/1(TestOk), Trq_2ms/3, SetNtcSts/3(NtcSts), DebStepSelection/1(TestOk)  "TestOk"
  HwTq3Polarity/1 -> PolarityEvaluation/2(HwTq3Polarity)
  NtcNr/1 -> SetNtcSts/1(NtcNr)  "NtcNr"
  PrtclFltEvln/3(ParamByte) -> SetNtcSts/2(NtcStInfo)  "ParamByte"
  NtcNr1/1 -> GetNtcQlfr/1(NtcNr)
  DebStepSelection/1(DebStep) -> SetNtcSts/4(DebStep)
  PolarityEvaluation/1(HwTq3) -> Trq_2ms/1, HwTq3/1  "HwTq3"
  RollCnt1/1(HwTq3RollgCntr) -> Unit Delay/1, Trq_2ms/2, HwTq3RollgCntr/1  "HwTq3RollgCntr"
  Unit Delay/1 -> RollCnt1/2(HwTq3PrevRollgCntr)
  NtcNr2/1 -> GetNtcQlfr1/1(NtcNr)
  GetNtcQlfr/1(NtcQlfr) -> If1/1
  GetNtcQlfr1/1(NtcQlfr) -> If1/2
  If Action Subsystem1/1(Qlfr) -> Merge1/1
  If Action Subsystem3/1(Qlfr) -> Merge1/2
  Merge1/1 -> Trq_2ms/4, HwTq3Qlfr/1  "HwTq3Qlfr"
  If1/2 -> If Action Subsystem3/Action
  If1/1 -> If Action Subsystem1/Action
  FCCNMASK_CNT_U32/1 -> PrtclFltEvln/3(HwTq3FCCN)
  TQDATAMASK_CNT_U32/1 -> PrtclFltEvln/4(HwTq3Data)
  RegInpRSENT5FRS/1 -> If/1
  If/1 -> Read the Flag/Action
  If/2 -> Do nothing/Action
  RegInpRSENT5FND/1 -> Read the Flag/1(RegInpRSENT5FND)
  ClearFlag/1 -> RegOutRSENT5CSC/1
  CSMASK_CNT_U32/1 -> Data Type Conversion1/1
  FRSMASK_CNT_U32/1 -> PrtclFltEvln/1(HwTq3FRS)
  Data Type Conversion1/1 -> PrtclFltEvln/2(HwTq3CS)
  RegInpRSENT5FRXD/1 -> SLOWNEWMSGDATAMASK_CNT_U32/1, TQDATAMASK_CNT_U32/1, FCCNMASK_CNT_U32/1
  RegInpRSENT5CS/1 -> SLOWCSMASK_ULS_U32/1, CSMASK_CNT_U32/1, FRSMASK_CNT_U32/1
  SlowSerlDataRead/1(GearIdn2Vld) -> GearIdn2Vld/1
  SlowSerlDataRead/2(GearIdn2) -> Saturation/1
  SLOWCSMASK_ULS_U32/1 -> SlowSerlDataRead/2(SlowSerlCS)
  SLOWNEWMSGDATAMASK_CNT_U32/1 -> SlowSerlDataRead/1(SlowSerlSND)
  RegInpRSENT5SRXD/1 -> SLOWMSGDATAMASK_CNT_U32/1, SLOWMSGIDMASK_CNT_U32/1
  SLOWMSGIDMASK_CNT_U32/1 -> RSHIFT8/1
  SLOWMSGDATAMASK_CNT_U32/1 -> Data Type Conversion3/1
  RSHIFT8/1 -> Data Type Conversion/1
  Data Type Conversion3/1 -> SlowSerlDataRead/4(SlowSerlMsgData)
  Data Type Conversion/1 -> SlowSerlDataRead/3(SlowSerlMsgID)
  Saturation/1 -> GearIdn2/1

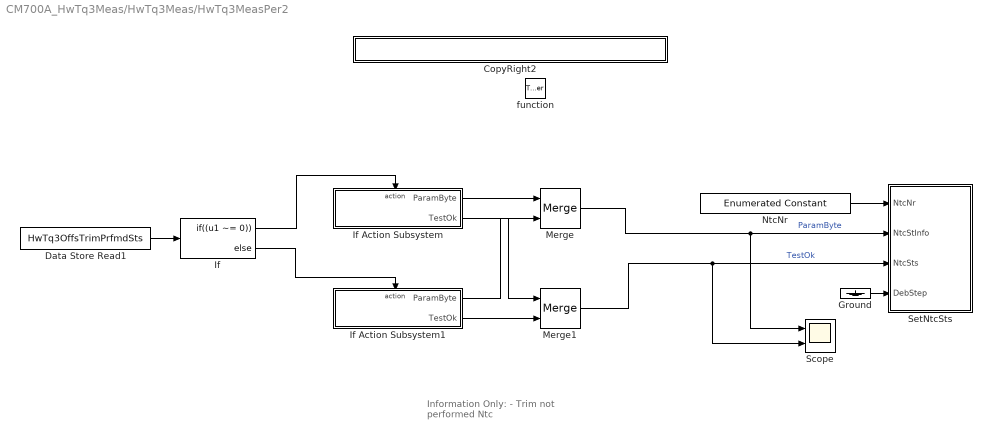
== system CM700A_HwTq3Meas/HwTq3Meas/HwTq3MeasPer2 ==
  note: Information Only:
      | - Trim not performed Ntc
  function : TriggerPort  TriggerType=function-call
  CopyRight2 : Subsystem  Description=|  mask(Copyright Information){none=on}
      | Copyright info block.                                               
      |                                                                     
      | Place copyright information at the top of every subsystem in design.
      mask prompts: none "No parameters"
      mask help: Place copyright information at the top of every subsystem in design.
      mask Display:
      | NxtrConf = 'Nexteer Confidential';
      | 
      | sys = bdroot; %handle for the current model ("system")
      | first = get_param(sys,'Created');
      | first = first(end-3:end);  %year is last four digits
      | 
      | last = get_param(sys,'LastModifiedDate');
      | if isempty(last)
      |     last = datestr(now,'yyyy');
      | else
      |     last = last(end-3:end);
      | end
      | 
      | if strcmp(first,last)
      |     fprintf('%s -- Copyright %s Nexteer',NxtrConf,first)
      | else
      |     fprintf('%s -- %s%s- %s Nexteer',NxtrConf,char(169),first,last)
      | end
  Data Store Read1 : DataStoreRead  DataStoreName=HwTq3OffsTrimPrfmdSts
  Ground : Ground
  If : If  IfExpression=(u1 ~= 0)
  If Action Subsystem : Subsystem  RequirementInfo={'linktype_rmi_doors' '0000cf43 (/ESG Group/FDD Module Requirements/EA4 Specific/CM700A_HwTq3Meas)' '#CM700A_65' 'true' 'REQ: CM700A_65' '' } %GIDa_eda0e9fe_0ef4_4d37_918c_815346a1604f  TreatAsAtomicUnit=on
  If Action Subsystem1 : Subsystem  RequirementInfo={'linktype_rmi_doors' '0000cf43 (/ESG Group/FDD Module Requirements/EA4 Specific/CM700A_HwTq3Meas)' '#CM700A_63' 'true' 'REQ: CM700A_63' '' } %GIDa_f1a05e9a_fff8_4eab_8b85_2e72f495a740  TreatAsAtomicUnit=on
  Merge : Merge
  Merge1 : Merge
  NtcNr : simulink/Sources/Enumerated Constant  OutDataTypeStr=Enum: NtcNr1  Value=NtcNr1.NTCNR_0X1E3  SampleTime=inf
  Scope : Scope  NumInputPorts=2
      settings: YMin=-5~-5  YMax=5~5  SaveName=ScopeData3
  SetNtcSts : Subsystem  RequirementInfo={'linktype_rmi_doors' '0000cf43 (/ESG Group/FDD Module Requirements/EA4 Specific/CM700A_HwTq3Meas)' '#CM700A_59' 'true' 'REQ: CM700A_59' '' } %GIDa_03dde2fd_062f_4b23_859a_fc5579118954
  wires:
  Ground/1 -> SetNtcSts/4(DebStep)
  NtcNr/1 -> SetNtcSts/1(NtcNr)
  Data Store Read1/1 -> If/1
  If/1 -> If Action Subsystem/Action
  If/2 -> If Action Subsystem1/Action
  If Action Subsystem/1(ParamByte) -> Merge/1
  If Action Subsystem1/1(ParamByte) -> Merge/2
  If Action Subsystem/2(TestOk) -> Merge1/1
  If Action Subsystem1/2(TestOk) -> Merge1/2
  Merge/1 -> Scope/1, SetNtcSts/2(NtcStInfo)  "ParamByte"
  Merge1/1 -> Scope/2, SetNtcSts/3(NtcSts)  "TestOk"

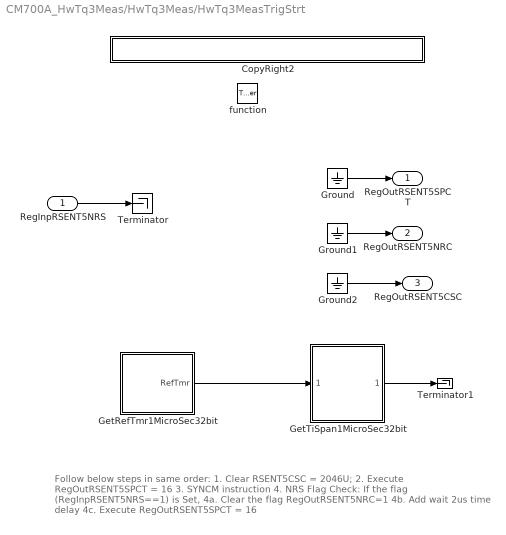
== system CM700A_HwTq3Meas/HwTq3Meas/HwTq3MeasTrigStrt ==
  note: Follow below steps in same order:
      |
      | 1. Clear RSENT5CSC = 2046U;
      | 2. Execute RegOutRSENT5SPCT = 16
      | 3. SYNCM instruction
      |
      | 4. NRS Flag Check: If the flag (RegInpRSENT5NRS==1) is Set,
      | 	4a. Clear the flag RegOutRSENT5NRC=1
      | 	4b. Add wait 2us time delay
      | 	4c. Execute RegOutRSENT5SPCT = 16
  RegInpRSENT5NRS : Inport
  function : TriggerPort  TriggerType=function-call
  CopyRight2 : Subsystem  Description=|  mask(Copyright Information){none=on}
      | Copyright info block.                                               
      |                                                                     
      | Place copyright information at the top of every subsystem in design.
      mask prompts: none "No parameters"
      mask help: Place copyright information at the top of every subsystem in design.
      mask Display:
      | NxtrConf = 'Nexteer Confidential';
      | 
      | sys = bdroot; %handle for the current model ("system")
      | first = get_param(sys,'Created');
      | first = first(end-3:end);  %year is last four digits
      | 
      | last = get_param(sys,'LastModifiedDate');
      | if isempty(last)
      |     last = datestr(now,'yyyy');
      | else
      |     last = last(end-3:end);
      | end
      | 
      | if strcmp(first,last)
      |     fprintf('%s -- Copyright %s Nexteer',NxtrConf,first)
      | else
      |     fprintf('%s -- %s%s- %s Nexteer',NxtrConf,char(169),first,last)
      | end
  GetRefTmr1MicroSec32bit : Subsystem
      settings: AttributesFormatString=Client Call : Start Time
  GetTiSpan1MicroSec32bit : Subsystem
  Ground : Ground
  Ground1 : Ground
  Ground2 : Ground
  Terminator : Terminator
  Terminator1 : Terminator
  RegOutRSENT5SPCT : Outport
  RegOutRSENT5NRC : Outport  Port=2
  RegOutRSENT5CSC : Outport  Port=3
  wires:
  Ground1/1 -> RegOutRSENT5NRC/1
  Ground/1 -> RegOutRSENT5SPCT/1
  Ground2/1 -> RegOutRSENT5CSC/1
  RegInpRSENT5NRS/1 -> Terminator/1
  GetTiSpan1MicroSec32bit/1(TiSpan) -> Terminator1/1
  GetRefTmr1MicroSec32bit/1(RefTmr) -> GetTiSpan1MicroSec32bit/1(RefTmr)

== system CM700A_HwTq3Meas/Simulated_Input/CopyRight2 ==

== system CM700A_HwTq3Meas/Simulated_Input/Signal Builder ==
  Demux : Demux  Tag=STV Demux  Outputs=8
  FromWs : FromWorkspace  Tag=STV FromWs  VariableName=tuvar  SampleTime=0  OutputAfterFinalValue=Holding final value
      SigBuilderData=|
      | common.afterFinalStr = 'Hold final value'
      | common.sampleTime = '0'
      | dataSet(1).timeRange = [0 20]
      | dataSet(1).name = 'IdealSignal'
      | dataSet(2).timeRange = [0 20]
      | dataSet(2).name = 'Faults'
      | dataSet(3).timeRange = [0 20]
      | dataSet(3).name = 'Service'
      | sbobj.Groups(1).Name = 'IdealSignal'
      | sbobj.Groups(1).Signals(1).Name = 'InitTrg'
      | sbobj.Groups(1).Signals(1).XData = [0 0.02 0.02 0.06 0.06 20]
      | sbobj.Groups(1).Signals(1).YData = [0 0 1 1 0 0]
      | sbobj.Groups(1).Signals(2).Name = 'AutTrimSrv'
      | sbobj.Groups(1).Signals(2).XData = [0 20]
      | sbobj.Groups(1).Signals(2).YData = [0 0]
      | sbobj.Groups(1).Signals(3).Name = 'ClearTrimSrv'
      | sbobj.Groups(1).Signals(3).XData = [0 20]
      | sbobj.Groups(1).Signals(3).YData = [0 0]
      | sbobj.Groups(1).Signals(4).Name = 'ReadTrimSrv'
      | sbobj.Groups(1).Signals(4).XData = [0 20]
      | sbobj.Groups(1).Signals(4).YData = [0 0]
      | sbobj.Groups(1).Signals(5).Name = 'WrSrv'
      | sbobj.Groups(1).Signals(5).XData = [0 0.04 0.04 0.08 0.08 20]
      | sbobj.Groups(1).Signals(5).YData = [0 0 1 1 0 0]
      | sbobj.Groups(1).Signals(6).Name = 'TrimPrfmdStsSrv'
      | sbobj.Groups(1).Signals(6).XData = [0 20]
      | sbobj.Groups(1).Signals(6).YData = [0 0]
      | sbobj.Groups(1).Signals(7).Name = 'HwTqOffsTrimData'
      | sbobj.Groups(1).Signals(7).XData = [0 20]
      | sbobj.Groups(1).Signals(7).YData = [0 0]
      | sbobj.Groups(1).Signals(8).Name = 'Polarity'
      | sbobj.Groups(1).Signals(8).XData = [0 20]
      | sbobj.Groups(1).Signals(8).YData = [1 1]
      | sbobj.Groups(1).TimeRange = [0 20]
      | sbobj.Groups(2).Name = 'Faults'
      | sbobj.Groups(2).Signals(1).Name = 'InitTrg'
      | sbobj.Groups(2).Signals(1).XData = [0 0.02 0.02 0.06 0.06 20]
      | sbobj.Groups(2).Signals(1).YData = [0 0 1 1 0 0]
      | sbobj.Groups(2).Signals(2).Name = 'AutTrimSrv'
      | sbobj.Groups(2).Signals(2).XData = [0 20]
      | sbobj.Groups(2).Signals(2).YData = [0 0]
      | sbobj.Groups(2).Signals(3).Name = 'ClearTrimSrv'
      | sbobj.Groups(2).Signals(3).XData = [0 20]
      | sbobj.Groups(2).Signals(3).YData = [0 0]
      | sbobj.Groups(2).Signals(4).Name = 'ReadTrimSrv'
      | sbobj.Groups(2).Signals(4).XData = [0 20]
      | sbobj.Groups(2).Signals(4).YData = [0 0]
      | sbobj.Groups(2).Signals(5).Name = 'WrSrv'
      | sbobj.Groups(2).Signals(5).XData = [0 0.06 0.06 0.12 0.12 20]
      | sbobj.Groups(2).Signals(5).YData = [0 0 1 1 0 0]
      | sbobj.Groups(2).Signals(6).Name = 'TrimPrfmdStsSrv'
      | sbobj.Groups(2).Signals(6).XData = [0 20]
      | sbobj.Groups(2).Signals(6).YData = [0 0]
      | sbobj.Groups(2).Signals(7).Name = 'HwTqOffsTrimData'
      | sbobj.Groups(2).Signals(7).XData = [0 20]
      | sbobj.Groups(2).Signals(7).YData = [0 0]
      | sbobj.Groups(2).Signals(8).Name = 'Polarity'
      | sbobj.Groups(2).Signals(8).XData = [0 11 11 20]
      | sbobj.Groups(2).Signals(8).YData = [-1 -1 1 1]
      | sbobj.Groups(2).TimeRange = [0 20]
      | sbobj.Groups(3).Name = 'Service'
      | sbobj.Groups(3).Signals(1).Name = 'InitTrg'
      | sbobj.Groups(3).Signals(1).XData = [0 0.02 0.02 0.06 0.06 20]
      | sbobj.Groups(3).Signals(1).YData = [0 0 1 1 0 0]
      | sbobj.Groups(3).Signals(2).Name = 'AutTrimSrv'
      | sbobj.Groups(3).Signals(2).XData = [0 0.58 0.58 0.68 0.68 16 16 16.1 16.1 20]
      | sbobj.Groups(3).Signals(2).YData = [0 0 1 1 0 0 1 1 0 0]
      | sbobj.Groups(3).Signals(3).Name = 'ClearTrimSrv'
      | sbobj.Groups(3).Signals(3).XData = [0 0.34 4.1 4.1 4.16 4.16 9.98 9.98 10.06 10.06 20]
      | sbobj.Groups(3).Signals(3).YData = [0 0 0 1 1 0 0 1 1 0 0]
      | sbobj.Groups(3).Signals(4).Name = 'ReadTrimSrv'
      | sbobj.Groups(3).Signals(4).XData = [0 1.24 1.24 1.32 1.32 4.62 4.62 4.7 4.7 6.84 6.84 6.92 6.92 10.38 10.38 10.46 10.46 16.72 16.72 16.8 16.8 20]
      | sbobj.Groups(3).Signals(4).YData = [0 0 1 1 0 0 1 1 0 0 1 1 0 0 1 1 0 0 1 1 0 0]
      | sbobj.Groups(3).Signals(5).Name = 'WrSrv'
      | sbobj.Groups(3).Signals(5).XData = [0 6.22 6.22 6.3 6.3 20]
      | sbobj.Groups(3).Signals(5).YData = [0 0 1 1 0 0]
      | sbobj.Groups(3).Signals(6).Name = 'TrimPrfmdStsSrv'
      | sbobj.Groups(3).Signals(6).XData = [0 1.24 1.24 1.32 1.32 4.64 4.64 4.7 4.7 6.84 6.84 6.92 6.92 10.64 10.64 10.72 10.72 16.74 16.74 16.82 16.82 20]
      | sbobj.Groups(3).Signals(6).YData = [0 0 1 1 0 0 1 1 0 0 1 1 0 0 1 1 0 0 1 1 0 0]
      | sbobj.Groups(3).Signals(7).Name = 'HwTqOffsTrimData'
      | sbobj.Groups(3).Signals(7).XData = [0 0.4 5.78 5.78 7.62 7.62 20]
      | sbobj.Groups(3).Signals(7).YData = [0 0 0 5 5 0 0]
      | sbobj.Groups(3).Signals(8).Name = 'Polarity'
      | sbobj.Groups(3).Signals(8).XData = [0 20]
      | sbobj.Groups(3).Signals(8).YData = [1 1]
      | sbobj.Groups(3).TimeRange = [0 20]
  InitTrg : Outport  Tag=STV Outport
  AutTrimSrv : Outport  Tag=STV Outport  Port=2
  ClearTrimSrv : Outport  Tag=STV Outport  Port=3
  ReadTrimSrv : Outport  Tag=STV Outport  Port=4
  WrSrv : Outport  Tag=STV Outport  Port=5
  TrimPrfmdStsSrv : Outport  Tag=STV Outport  Port=6
  HwTqOffsTrimData : Outport  Tag=STV Outport  Port=7
  Polarity : Outport  Tag=STV Outport  Port=8
  wires:
  Demux/8 -> Polarity/1
  Demux/7 -> HwTqOffsTrimData/1
  Demux/6 -> TrimPrfmdStsSrv/1
  Demux/5 -> WrSrv/1
  Demux/4 -> ReadTrimSrv/1
  Demux/3 -> ClearTrimSrv/1
  Demux/2 -> AutTrimSrv/1
  Demux/1 -> InitTrg/1
  FromWs/1 -> Demux/1

== system CM700A_HwTq3Meas/HwTq3Meas/HwTq3MeasHwTq3AutTrim/CopyRight2 ==

== system CM700A_HwTq3Meas/HwTq3Meas/HwTq3MeasHwTq3ClrTrim/CopyRight2 ==

== system CM700A_HwTq3Meas/HwTq3Meas/HwTq3MeasHwTq3ReadTrim/CopyRight2 ==

== system CM700A_HwTq3Meas/HwTq3Meas/HwTq3MeasHwTq3TrimPrfmdSts/CopyRight2 ==

== system CM700A_HwTq3Meas/HwTq3Meas/HwTq3MeasHwTq3WrTrim/CopyRight2 ==

== system CM700A_HwTq3Meas/HwTq3Meas/HwTq3MeasInit1/CopyRight2 ==
